simulink model "gm_ifft_16_bit"  (R2016b)
settings: Solver=FixedStepDiscrete  StartTime=0.0  StopTime=10.0  RelTol=1e-3
libraries: dspxfrm3 x1
settings Model: Creator=mw  LastModifiedBy=mw
settings DataIOCC: SaveOutput=off  SaveTime=off
settings OptimizationCC: BlockReduction=off  ConditionallyExecuteInputs=off  DefaultParameterBehavior=Inlined
settings DebuggingCC: AlgebraicLoopMsg=error  InheritedTsInSrcMsg=none  SingleTaskRateTransMsg=error  StrictBusMsg=ErrorOnBusTreatedAsVector
settings HardwareCC: ProdBitPerPointer=32  ProdBitPerSizeT=32  ProdBitPerPtrDiffT=32  ProdLargestAtomicFloat=None  ProdIntDivRoundTo=Undefined  ProdEndianess=Unspecified  ProdWordSize=32  ProdHWDeviceType=ASIC/FPGA->ASIC/FPGA  ProdEqTarget=off
settings GRTTargetCC: TargetLangStandard=C89/C90 (ANSI)

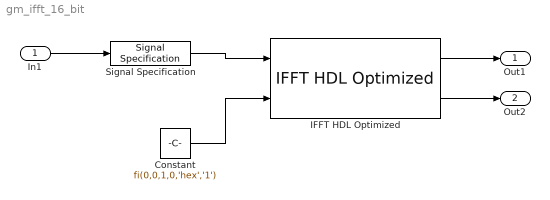
== system gm_ifft_16_bit ==
  In1 : Inport  OutDataTypeStr=uint16  PortDimensions=[16]  SampleTime=0.2
  Constant : Constant  Value=fi(0,0,1,0,'hex','1')  OutDataTypeStr=boolean  SampleTime=-1
  IFFT HDL Optimized : dspxfrm3/IFFT HDL Optimized  Architecture=Streaming Radix 2^2  ComplexMultiplication=Use 3 multipliers and 5 adders  BitReversedOutput=on  BitReversedInput=off  Normalize=on  FFTLength=16  SimulateUsing=Code generation  RoundingMethod=Floor  ResetInputPort=off  StartOutputPort=off  EndOutputPort=off
  Signal Specification : SignalSpecification  OutDataTypeStr=uint16  Dimensions=16
  Out1 : Outport
  Out2 : Outport  Port=2
  wires:
  In1/1 -> Signal Specification/1
  Constant/1 -> IFFT HDL Optimized/2
  IFFT HDL Optimized/1 -> Out1/1
  IFFT HDL Optimized/2 -> Out2/1
  Signal Specification/1 -> IFFT HDL Optimized/1
